simulink model "ZT_VehCtrl_18B"  (R2018b)
settings: Solver=FixedStepAuto  StartTime=0.0  StopTime=inf  FixedStep=0.005  RelTol=1e-3
InitFcn:
  | mbd_mpc_consistency_checks(bdroot(gcs));
undefined symbols (not defined in the file or in its folder): ANG_DEAD, BMS_NormalPwr, BrkPrsByBrkPct_TB_X, BrkPrsByBrkPct_TB_Y, DELAY_DISCHARGE, DELAY_RCUOFF, DRV_BACKWARD, DRV_BRAKE, DRV_FORWARD, DRV_NEUTRAL, DRV_PARK, DRV_UNPARK, DRV_ZEROTURN, EPB_LOCK, EPB_UNLOCK, ExtraLoadPwr, FanOff, fifo_0_vect, fifo_1_vect, HiFanReq, HV_finished, HV_No_Active, HV_POWER_OFF, HV_POWER_ON, HVDown, HVON, KaTLS_v_DrgUp_X_VehSpd, KeFTM_s_Way1OffDlyTime, KeFTM_TK_Way1CoolLv2OffBatTemp, KeFTM_TK_Way1CoolLv2OffMtrTemp, KeFTM_TK_Way1CoolLv2OnBatTemp, KeFTM_TK_Way1CoolLv2OnMtrTemp, KeFTM_TK_Way1CoolLv3OffBatTemp, KeFTM_TK_Way1CoolLv3OffMtrTemp, KeFTM_TK_Way1CoolLv3OnBatTemp, KeFTM_TK_Way1CoolLv3OnMtrTemp, KeFTM_TK_Way1CoolLv4OffBatTemp, KeFTM_TK_Way1CoolLv4OffMtrTemp, KeFTM_TK_Way1CoolLv4OnBatTemp, KeFTM_TK_Way1CoolLv4OnMtrTemp, Kp1, Kp2, LowFanReq, LQFP, MtrPwrFactor_RCU, MtrPwrHighToMidThd, MtrPwrLowToMidThd, MtrPwrMidToHighThd, MtrPwrMidToLowThd, MtrTrqMax, PCT_DEAD, Precharge, PTO_1000, PTO_540, pts1_fifo_0_vect, pts1_fifo_1_vect, pts2_fifo_0_vect, pts2_fifo_1_vect, pts3_fifo_0_vect, pts3_fifo_1_vect ... (+24)
libraries: mbd_mpc574x_ec_toolbox x173, canmsglib x72, simulink x57
(part 6 of 12)

== system ZT_VehCtrl_18B/SigOut/GPIO /HS ==
  note: 3A/5A
  note: 1A/3A
  note: 0.5A/1A
  Data Store Read : DataStoreRead  DataStoreName=HS001
  Data Store Read2 : DataStoreRead  DataStoreName=HS007
  Data Store Read4 : DataStoreRead  DataStoreName=HS002
  Data Store Read5 : DataStoreRead  DataStoreName=HS003
  Data Store Read6 : DataStoreRead  DataStoreName=HS004
  Data Store Read7 : DataStoreRead  DataStoreName=HS005
  Data Store Read9 : DataStoreRead  DataStoreName=HS010
  HS001 : mbd_mpc574x_ec_toolbox/GPIO Blocks/Digital_Output  Priority=1  gpio_pin=PTF5: [SIUL2_GPIO85 | General Purpose IO PF[5]]  gpio_drive_strength=Disabled
  "HS002 " : mbd_mpc574x_ec_toolbox/GPIO Blocks/Digital_Output  Priority=1  gpio_pin=PTF4: [SIUL2_GPIO84 | General Purpose IO PF[4]]  gpio_drive_strength=Disabled
  HS003 : mbd_mpc574x_ec_toolbox/GPIO Blocks/Digital_Output  Priority=1  gpio_pin=PTF3: [SIUL2_GPIO83 | General Purpose IO PF[3]]  gpio_drive_strength=Disabled
  HS004 : mbd_mpc574x_ec_toolbox/GPIO Blocks/Digital_Output  Priority=1  gpio_pin=PTB6: [SIUL2_GPIO22 | General Purpose IO PB[6]]  gpio_drive_strength=Disabled
  HS005 : mbd_mpc574x_ec_toolbox/GPIO Blocks/Digital_Output  Priority=1  gpio_pin=PTA12: [SIUL2_GPIO12 | General Purpose IO PA[12]]  gpio_drive_strength=Disabled
  HS007 : mbd_mpc574x_ec_toolbox/GPIO Blocks/Digital_Output  Priority=1  gpio_pin=PTF7: [SIUL2_GPIO87 | General Purpose IO PF[7]]  gpio_drive_strength=Disabled
  HS010 : mbd_mpc574x_ec_toolbox/GPIO Blocks/Digital_Output  Priority=1  gpio_pin=PTF9: [SIUL2_GPIO89 | General Purpose IO PF[9]]  gpio_drive_strength=Disabled
  wires:
  Data Store Read/1 -> HS001/1
  Data Store Read5/1 -> HS003/1
  Data Store Read4/1 -> "HS002 "/1
  Data Store Read6/1 -> HS004/1
  Data Store Read7/1 -> HS005/1
  Data Store Read2/1 -> HS007/1
  Data Store Read9/1 -> HS010/1

== system ZT_VehCtrl_18B/SigOut/GPIO /PWM_OUT ==
  note: LS PWM
  note: HS PWM
  note: Example
  Data Store Read10 : DataStoreRead  DataStoreName=HSO14_PWM_DC
  Data Store Read11 : DataStoreRead  DataStoreName=HSO14_PWM_FRQ
  Data Store Read14 : DataStoreRead  DataStoreName=LSO19_PWM_DC
  Data Store Read15 : DataStoreRead  DataStoreName=LSO19_PWM_FRQ
  Data Store Read2 : DataStoreRead  DataStoreName=HSO08_PWM_DC
  Data Store Read9 : DataStoreRead  DataStoreName=HSO08_PWM_FRQ
  FreqCMD : Stateflow chart  Priority=0  Commented=on  TreatAsAtomicUnit=on
  PWM Configuration and Frequency Update : Subsystem  Commented=on
  PWM Configuration and Frequency Update1 : Subsystem
  PWM Configuration and Frequency Update4 : Subsystem
  wires:
  FreqCMD/1(freq) -> PWM Configuration and Frequency Update/1(In1)
  FreqCMD/2(dc) -> PWM Configuration and Frequency Update/2(In2)
  Data Store Read9/1 -> PWM Configuration and Frequency Update1/2(Fre A)
  Data Store Read2/1 -> PWM Configuration and Frequency Update1/1(PWM A)
  Data Store Read14/1 -> PWM Configuration and Frequency Update4/1(PWM A)
  Data Store Read10/1 -> PWM Configuration and Frequency Update1/3(PWM B)
  Data Store Read11/1 -> PWM Configuration and Frequency Update1/4(Fre B)
  Data Store Read15/1 -> PWM Configuration and Frequency Update4/2(Fre)

== system ZT_VehCtrl_18B/SigOut/GPIO /SPI0: LS09_14_15_16_1_2_11_4 ==
  note: 不要开，会重置SPI的初始化设置
  Compare To Constant : simulink/Logic and Bit Operations/Compare To Constant  relop===  const=2  OutDataTypeStr=boolean
  Constant : Constant  OutDataTypeStr=boolean
  Constant1 : Constant  OutDataTypeStr=boolean
  Constant2 : Constant  OutDataTypeStr=boolean
  Data Store Read : DataStoreRead  DataStoreName=VCU_Mode
  Data Store Read1 : DataStoreRead  DataStoreName=SPI0_CS
  LS_CTRL : Subsystem
  LS_CTRL1 : Subsystem
  LS_EN : mbd_mpc574x_ec_toolbox/GPIO Blocks/Digital_Output  Priority=1  gpio_pin=PTA2: [SIUL2_GPIO2 | General Purpose IO PA[2]]  gpio_drive_strength=Disabled
  LS_rst1 : mbd_mpc574x_ec_toolbox/GPIO Blocks/Digital_Output  Priority=1  gpio_pin=PTC10: [SIUL2_GPIO42 | General Purpose IO PC[10]]  gpio_drive_strength=Disabled
  LS_rst2 : mbd_mpc574x_ec_toolbox/GPIO Blocks/Digital_Output  Priority=1  gpio_pin=PTA1: [SIUL2_GPIO1 | General Purpose IO PA[1]]  gpio_drive_strength=Disabled
  Logical Operator : Logic  AllPortsSameDT=off  OutDataTypeStr=boolean
  Logical Operator1 : Logic  Operator=NOT  AllPortsSameDT=off  OutDataTypeStr=boolean
  wires:
  Constant1/1 -> LS_rst2/1
  Constant/1 -> LS_EN/1
  Constant2/1 -> LS_rst1/1
  Data Store Read/1 -> Compare To Constant/1
  Compare To Constant/1 -> Logical Operator/1
  Data Store Read1/1 -> Logical Operator/2
  Logical Operator/1 -> LS_CTRL1/Enable, Logical Operator1/1
  Logical Operator1/1 -> LS_CTRL/Enable

== system ZT_VehCtrl_18B/SigOut/GPIO /SPI3: LS03_06_07_08_10_12_13_17_18_19 ==
  Compare To Constant : simulink/Logic and Bit Operations/Compare To Constant  relop===  const=2  OutDataTypeStr=boolean
  Constant1 : Constant  OutDataTypeStr=boolean
  Constant3 : Constant  OutDataTypeStr=boolean
  Data Store Read : DataStoreRead  DataStoreName=VCU_Mode
  Data Store Read3 : DataStoreRead  DataStoreName=SPI3_CS
  LS_EN1 : mbd_mpc574x_ec_toolbox/GPIO Blocks/Digital_Output  Priority=1  gpio_pin=PTF10: [SIUL2_GPIO90 | General Purpose IO PF[10]]  gpio_drive_strength=Disabled
  LS_rst : mbd_mpc574x_ec_toolbox/GPIO Blocks/Digital_Output  Priority=1  gpio_pin=PTC14: [SIUL2_GPIO46 | General Purpose IO PC[14]]  gpio_drive_strength=Disabled
  Logical Operator : Logic  AllPortsSameDT=off  OutDataTypeStr=boolean
  Subsystem : Subsystem
  wires:
  Constant1/1 -> LS_EN1/1
  Constant3/1 -> LS_rst/1
  Data Store Read/1 -> Compare To Constant/1
  Data Store Read3/1 -> Logical Operator/2
  Compare To Constant/1 -> Logical Operator/1
  Logical Operator/1 -> Subsystem/Enable

== system ZT_VehCtrl_18B/VehCtrl/EnergyManage1/Subsystem ==
  VehTrqTgt : Inport
  VehSpd : Inport  Port=2
  MCU_PTO : Inport  Port=3
  Add : Sum
  Bus Selector3 : BusSelector  OutputSignals=MCU2VCU_1.MCU_TrqEst,MCU2VCU_1.MCU_SpdEst
  Constant2 : Constant  Value=WhlRadius
  Constant3 : Constant  Value=9.55  OutDataTypeStr=single
  Divide : Product  Inputs=*/
  Divide1 : Product  Inputs=*/
  Product : Product
  Product1 : Product
  PwrCmd : Outport
  wires:
  Constant3/1 -> Divide1/2
  Divide/1 -> Product/2
  Product/1 -> Add/1
  Constant2/1 -> Divide/2
  Bus Selector3/2 -> Divide1/1  "<MCU_SpdEst>"
  Divide1/1 -> Product1/2
  Product1/1 -> Add/2
  Bus Selector3/1 -> Product1/1  "<MCU_TrqEst>"
  VehTrqTgt/1 -> Product/1
  VehSpd/1 -> Divide/1
  Add/1 -> PwrCmd/1
  MCU_PTO/1 -> Bus Selector3/1

== system ZT_VehCtrl_18B/VehCtrl/FaultProc/Subsystem5 ==
  note: 1-正常
      | 0-超时
  note: 1-丢包
      | 0-正常
  AutoDrive : Inport
  Bus Selector7 : BusSelector  OutputSignals=signal1.AUTO_LiveCnt1,signal1.AUTO_CheckSum1,signal1.PacketLossFlg,signal2.AUTO_LiveCnt2,signal2.AUTO_CheckSum2,signal2.PacketLossFlg,signal3.AUTO_LiveCnt1,signal3.AUTO_CheckSum1,signal3.PacketLossFlg
  Logical Operator : Logic  Operator=NOT  AllPortsSameDT=off  OutDataTypeStr=boolean
  Logical Operator1 : Logic  Operator=OR  Inputs=3  AllPortsSameDT=off  OutDataTypeStr=boolean
  Logical Operator2 : Logic  Inputs=3  AllPortsSameDT=off  OutDataTypeStr=boolean
  PacketLoss_RMT : Stateflow chart  TreatAsAtomicUnit=on
  PacketLoss_RMT1 : Stateflow chart  TreatAsAtomicUnit=on
  PacketLoss_RMT2 : Stateflow chart  TreatAsAtomicUnit=on
  TimeOutLevel_RMT : Stateflow chart  TreatAsAtomicUnit=on
  TimeOutLevel_RMT1 : Stateflow chart  TreatAsAtomicUnit=on
  TimeOutLevel_RMT2 : Stateflow chart  TreatAsAtomicUnit=on
  TimeOut : Outport
  PacketLoss : Outport  Port=2
  wires:
  TimeOutLevel_RMT/1(TimeOutLevel) -> Logical Operator2/1  "TimeOutLevel1"
  Logical Operator2/1 -> Logical Operator/1
  [Auto_LiveCounter] -> TimeOutLevel_RMT/1(LiveCounter)
  Logical Operator1/1 -> PacketLoss/1
  [Auto_PacketLossFlg] -> PacketLoss_RMT/2(PacketLoss)
  [Auto_CheckSumFlg] -> PacketLoss_RMT/1(CheckSum)
  PacketLoss_RMT/1(PacketLossFlg) -> Logical Operator1/1
  AutoDrive/1 -> Bus Selector7/1
  Logical Operator/1 -> TimeOut/1
  [Auto_LiveCounter2] -> TimeOutLevel_RMT1/1(LiveCounter)
  TimeOutLevel_RMT1/1(TimeOutLevel) -> Logical Operator2/2  "TimeOutLevel1"
  [Auto_CheckSumFlg2] -> PacketLoss_RMT1/1(CheckSum)
  [Auto_PacketLossFlg2] -> PacketLoss_RMT1/2(PacketLoss)
  PacketLoss_RMT1/1(PacketLossFlg) -> Logical Operator1/2
  Bus Selector7/6 -> [Auto_PacketLossFlg2]  "<PacketLossFlg>"
  Bus Selector7/5 -> [Auto_CheckSumFlg2]  "<AUTO_CheckSum2>"
  Bus Selector7/4 -> [Auto_LiveCounter2]  "<AUTO_LiveCnt2>"
  Bus Selector7/3 -> [Auto_PacketLossFlg]  "<PacketLossFlg>"
  Bus Selector7/2 -> [Auto_CheckSumFlg]  "<AUTO_CheckSum1>"
  Bus Selector7/1 -> [Auto_LiveCounter]  "<AUTO_LiveCnt1>"
  Bus Selector7/7 -> [Auto_LiveCounter3]  "<AUTO_LiveCnt1>"
  Bus Selector7/8 -> [Auto_CheckSumFlg3]  "<AUTO_CheckSum1>"
  Bus Selector7/9 -> [Auto_PacketLossFlg3]  "<PacketLossFlg>"
  [Auto_LiveCounter3] -> TimeOutLevel_RMT2/1(LiveCounter)
  TimeOutLevel_RMT2/1(TimeOutLevel) -> Logical Operator2/3  "TimeOutLevel1"
  [Auto_PacketLossFlg3] -> PacketLoss_RMT2/2(PacketLoss)
  [Auto_CheckSumFlg3] -> PacketLoss_RMT2/1(CheckSum)
  PacketLoss_RMT2/1(PacketLossFlg) -> Logical Operator1/3

== system ZT_VehCtrl_18B/VehCtrl/MontionControl/DriveControl ==
  EN_COM : Inport
  Ready : Inport  Port=2
  Fault : Inport  Port=3
  CMD : Inport  Port=4
  BMS : Inport  Port=5
  VehSpd : Inport  Port=6
  StrReady : Inport  Port=7
  AUTO : Inport  Port=8
  AUTOMode : Inport  Port=9
  RMT : Inport  Port=10
  DCDC : Inport  Port=11
  Brake : Subsystem
  Bus Creator{1..4} (4 alike) : BusCreator  Inputs=4
  Bus Selector : BusSelector  OutputSignals=RMT.RMT1.RMT_CmdAccPct,BrkPct,ModeDir,ModeStr,StrAng,RMT.RMT4.ModeSafety
  Constant : Constant  Value=0  OutDataTypeStr=uint8
  Constant1 : Constant
  Constant2 : Constant  Value=0  OutDataTypeStr=uint8
  Constant3 : Constant  OutDataTypeStr=boolean
  DriveModeTrans : Stateflow chart  TreatAsAtomicUnit=on
  Equal : RelationalOperator  Operator===  OutDataTypeStr=boolean  RndMeth=Simplest
  Logical Operator : Logic  AllPortsSameDT=off  OutDataTypeStr=boolean
  Motor : Subsystem
  MCUFL_OUT : Outport
  MCUFR_OUT : Outport  Port=2
  MCURL_OUT : Outport  Port=3
  MCURR_OUT : Outport  Port=4
  BrkPrsTgt : Outport  Port=5
  EpbSt : Outport  Port=6
  VehTrqTgt : Outport  Port=7
  wires:
  CMD/1 -> Bus Selector/1
  Bus Selector/3 -> DriveModeTrans/5(ModeDirection)  "<ModeDir>"
  Bus Selector/2 -> DriveModeTrans/2(CmdBrk)  "<BrkPct>"
  Brake/1(BrkPrsTgt) -> BrkPrsTgt/1
  DriveModeTrans/1(VehBrk) -> Brake/1(VehBrkTgt)
  DriveModeTrans/2(EpbSt) -> EpbSt/1
  VehSpd/1 -> DriveModeTrans/9(VehSpd), Motor/5(VehSpd)
  DriveModeTrans/3(VehDrv) -> Motor/1(VehDrvPct)
  Bus Selector/1 -> DriveModeTrans/1(CmdDrv)  "<RMT_CmdAccPct>"
  Bus Selector/4 -> Logical Operator/1  "<ModeStr>"
  StrReady/1 -> DriveModeTrans/8(StrReady)
  DriveModeTrans/4(SpdTgt) -> Motor/2(CmdSpd)
  DriveModeTrans/5(ModeSpd) -> Motor/3(ModeSpeed)
  DriveModeTrans/6(DrvPhase) -> Motor/4(DrvPhase)
  Bus Selector/5 -> Motor/6(CmdStrAng)  "<StrAng>"
  Motor/2(MtrDirCmdFL) -> Bus Creator1/2  "DirCmd"
  Motor/1(Enable) -> Bus Creator1/1, Bus Creator2/1, Bus Creator4/1, Bus Creator3/1  "Enable"
  Bus Creator4/1 -> MCURR_OUT/1
  Bus Creator2/1 -> MCUFR_OUT/1
  Motor/13(MtrSpdCmdRR) -> Bus Creator4/4  "SpdCmd"
  Motor/12(MtrTrqCmdRR) -> Bus Creator4/3  "TrqCmd"
  Motor/11(MtrDirCmdRR) -> Bus Creator4/2  "DirCmd"
  Bus Creator1/1 -> MCUFL_OUT/1
  Motor/7(MtrSpdCmdFR) -> Bus Creator2/4  "SpdCmd"
  Motor/6(MtrTrqCmdFR) -> Bus Creator2/3  "TrqCmd"
  Bus Creator3/1 -> MCURL_OUT/1
  Motor/10(MtrSpdCmdRL) -> Bus Creator3/4  "SpdCmd"
  Motor/4(MtrSpdCmdFL) -> Bus Creator1/4  "SpdCmd"
  Motor/9(MtrTrqCmdRL) -> Bus Creator3/3  "TrqCmd"
  Motor/3(MtrTrqCmdFL) -> Bus Creator1/3  "TrqCmd"
  Motor/8(MtrDirCmdRL) -> Bus Creator3/2  "DirCmd"
  Motor/5(MtrDirCmdFR) -> Bus Creator2/2  "DirCmd"
  Ready/1 -> Motor/9(Ready)
  Motor/14(VehTrqTgt) -> VehTrqTgt/1
  Constant/1 -> DriveModeTrans/3(ModeDrive)
  Constant1/1 -> DriveModeTrans/4(CmdPark)
  Constant2/1 -> DriveModeTrans/7(CmdSpd)
  Bus Selector/6 -> Equal/1, Motor/7(ModeSafety)  "<ModeSafety>"
  AUTO/1 -> Motor/10(AUTO)
  AUTOMode/1 -> Motor/11(AUTOMode)
  BMS/1 -> Motor/12(BMS)
  RMT/1 -> Motor/13(RMT)
  DCDC/1 -> Motor/14(DCDC)
  Fault/1 -> Brake/2(In2), Motor/8(Fault)
  Logical Operator/1 -> DriveModeTrans/6(ModeSteer)
  Equal/1 -> Logical Operator/2
  Constant3/1 -> Equal/2
  EN_COM/1 -> Motor/15(EN_COM)

== system ZT_VehCtrl_18B/VehCtrl/MontionControl/PtoControl ==
  CMD : Inport
  Fault : Inport  Port=2
  Ready : Inport  Port=3
  AUTOMode : Inport  Port=4
  AUTO : Inport  Port=5
  Bus Creator : BusCreator  Inputs=4
  Bus Selector : BusSelector  OutputSignals=ShutDown,NonDrive,NonPto
  Bus Selector1 : BusSelector  OutputSignals=RMT.RMT4.RMT_PtoMode
  Bus Selector2 : BusSelector  OutputSignals=signal2.AUTO_PtoSpd
  Constant5 : Constant  Value=0  OutDataTypeStr=single
  Constant6 : Constant  OutDataTypeStr=uint8
  Constant7 : Constant  Value=0  OutDataTypeStr=uint8
  Logical Operator : Logic  Operator=OR  Inputs=3  AllPortsSameDT=off  OutDataTypeStr=boolean
  Logical Operator1 : Logic  AllPortsSameDT=off  OutDataTypeStr=boolean
  NOT : Logic  Operator=NOT  IconShape=distinctive  AllPortsSameDT=off  OutDataTypeStr=boolean
  Subsystem : Subsystem
  Subsystem1 : Subsystem
  Switch2 : Switch  Criteria=u2 > Threshold
  MCU_PTO_OUT : Outport
  wires:
  CMD/1 -> Bus Selector1/1
  Constant5/1 -> Bus Creator/3  "MtrTrqCmd"
  Subsystem/1(ModeReq) -> Bus Creator/1  "ModeReq"
  Constant6/1 -> Subsystem/1(ModeSpeed)
  Constant7/1 -> Subsystem/2(DirCmd)
  Fault/1 -> Bus Selector/1
  Bus Selector/1 -> Logical Operator/1  "<ShutDown>"
  Bus Selector/2 -> Logical Operator/2  "<NonDrive>"
  Bus Selector/3 -> Logical Operator/3  "<NonPto>"
  Logical Operator/1 -> NOT/1
  Ready/1 -> Logical Operator1/2
  NOT/1 -> Logical Operator1/1
  Logical Operator1/1 -> Bus Creator/4  "Enable"
  Bus Creator/1 -> MCU_PTO_OUT/1
  AUTOMode/1 -> Switch2/2
  Bus Selector1/1 -> Subsystem1/1(<RMT_PtoMode>)  "<RMT_PtoMode>"
  AUTO/1 -> Bus Selector2/1
  Bus Selector2/1 -> Switch2/1  "<AUTO_PtoSpd>"
  Switch2/1 -> Bus Creator/2  "MtrSpdCmd"
  Subsystem1/1(MtrSpdCmd) -> Switch2/3

== system ZT_VehCtrl_18B/VehCtrl/MontionControl/SteerControl ==
  note: 这个是模式，不是方向
  VehSpd : Inport
  CMD : Inport  Port=2
  BDX : Inport  Port=3
  Bus Selector : BusSelector  OutputSignals=ModeStr,StrAng
  Bus Selector1 : BusSelector  OutputSignals=AVCU.BDX_SteeringAngle
  Chart : Stateflow chart  TreatAsAtomicUnit=on
  Constant2 : Constant  Value=10  OutDataTypeStr=uint8
  GreaterThan : RelationalOperator  Operator=<  OutDataTypeStr=boolean  RndMeth=Simplest
  StrReady : Outport
  AngCmd : Outport  Port=2
  wires:
  CMD/1 -> Bus Selector/1
  Bus Selector/1 -> Chart/2(Mode)  "<ModeStr>"
  Bus Selector/2 -> Chart/3(AngCmd)  "<StrAng>"
  BDX/1 -> Bus Selector1/1
  Bus Selector1/1 -> Chart/4(Ang)  "<BDX_SteeringAngle>"
  Chart/2(StrPhase) -> GreaterThan/1
  GreaterThan/1 -> StrReady/1
  Constant2/1 -> GreaterThan/2
  VehSpd/1 -> Chart/1(VehSpd)
  Chart/1(AngCmdOut) -> AngCmd/1

== system ZT_VehCtrl_18B/VehCtrl/MontionControl/ValveControl ==
  note: 仅在安全模式下才能控制
  BrkPrsTgt : Inport
  EpbSt : Inport  Port=2
  BDX : Inport  Port=3
  CMD : Inport  Port=4
  Ready : Inport  Port=5
  "AngCmd " : Inport  Port=6
  fault : Inport  Port=7
  VehSpd : Inport  Port=8
  BrakeSys : Subsystem
  Bus Creator : BusCreator  Inputs=9
  Bus Selector : BusSelector  OutputSignals=ModeSusp,RMT.RMT4.ModeSafety,RMT.RMT2.RMT_ModeWidth
  Bus Selector1 : BusSelector  OutputSignals=AVCU.BDX_BrakePressure
  Bus Selector2 : BusSelector  OutputSignals=NonDrive
  EpbSys : Subsystem
  PumpSys : Subsystem
  SteerSys : Subsystem
  SuspesionSys : Subsystem
  WidthSys : Subsystem
  BDX_OUT : Outport
  wires:
  CMD/1 -> Bus Selector/1
  BDX/1 -> Bus Selector1/1
  BrkPrsTgt/1 -> BrakeSys/1(BrkPrsTgt)
  Bus Selector1/1 -> BrakeSys/2(BrkPrs)  "<BDX_BrakePressure>"
  Bus Selector/1 -> SuspesionSys/1(SuspSt)  "<ModeSusp>"
  Bus Selector/3 -> WidthSys/2(<RMT_ModeWidth>)  "<RMT_ModeWidth>"
  BrakeSys/1(BrkValve) -> Bus Creator/2  "BrkValve"
  SuspesionSys/1(SuspUpValve) -> Bus Creator/6  "SuspUpValve"
  PumpSys/1(Pump) -> Bus Creator/1  "Pump"
  EpbSys/1(EpbValve) -> Bus Creator/5  "EpbValve"
  SteerSys/1(SteerValveL) -> Bus Creator/3  "SteerValveL"
  WidthSys/1(WidthLengthenValve) -> Bus Creator/8  "WidthLengthenValve"
  WidthSys/2(WidthShortenValve) -> Bus Creator/9  "WidthShortenValve"
  Bus Creator/1 -> BDX_OUT/1
  SteerSys/2(SteerValveR) -> Bus Creator/4  "SteerValveR"
  EpbSt/1 -> EpbSys/1(EpbSt)
  SuspesionSys/2(SuspDownValve) -> Bus Creator/7  "SuspDownValve"
  Ready/1 -> PumpSys/1(Ready)
  Bus Selector/2 -> WidthSys/1(ModeSafety), SuspesionSys/2(ModeSafety)  "<ModeSafety>"
  fault/1 -> Bus Selector2/1
  Bus Selector2/1 -> SteerSys/2(In2)  "<NonDrive>"
  VehSpd/1 -> SteerSys/3(VehSpd)
  "AngCmd "/1 -> SteerSys/1(AngCmd)

== system ZT_VehCtrl_18B/VehCtrl/TempertureControl/Lv_to_Dut1 ==
  note: 就是整型，不要替换为single
  MCUReqMtrPumpLv : Inport
  2-D Lookup Table1 : Lookup_n-D  NumberOfTableDimensions=1  BreakpointsForDimension1=uint8([ 0 1 2 3 4 ])  BreakpointsForDimension2=KaTLS_v_DrgUp_X_VehSpd  Table=uint16([ 5 30 40 55 70])  TableDataTypeStr=uint16  ExtrapMethod=Clip  UseLastTableValue=on  OutDataTypeStr=Inherit: Inherit from 'Table data'  RndMeth=Simplest
  Gain : Gain  Gain=1/100  OutDataTypeStr=single
  MCUReqMtrPumpDut : Outport
  wires:
  MCUReqMtrPumpLv/1 -> 2-D Lookup Table1/1
  2-D Lookup Table1/1 -> Gain/1
  Gain/1 -> MCUReqMtrPumpDut/1

== system ZT_VehCtrl_18B/VehCtrl/TempertureControl/Lv_to_Dut2 ==
  note: 就是整型，不要替换为single
  MCUReqMtrPumpLv : Inport
  2-D Lookup Table1 : Lookup_n-D  NumberOfTableDimensions=1  BreakpointsForDimension1=uint8([ 0 1 2 3 4 ])  BreakpointsForDimension2=KaTLS_v_DrgUp_X_VehSpd  Table=uint16([ 5 30 40 55 70])  TableDataTypeStr=uint16  ExtrapMethod=Clip  UseLastTableValue=on  OutDataTypeStr=Inherit: Inherit from 'Table data'  RndMeth=Simplest
  Gain : Gain  Gain=1/100  OutDataTypeStr=single
  MCUReqMtrPumpDut : Outport
  wires:
  MCUReqMtrPumpLv/1 -> 2-D Lookup Table1/1
  2-D Lookup Table1/1 -> Gain/1
  Gain/1 -> MCUReqMtrPumpDut/1

== system ZT_VehCtrl_18B/VehCtrl/TempertureControl/Lv_to_Dut3 ==
  note: 就是整型，不要替换为single
  MCUReqBatPumpLv : Inport
  2-D Lookup Table1 : Lookup_n-D  NumberOfTableDimensions=1  BreakpointsForDimension1=uint8([ 0 1 2 3 4 ])  BreakpointsForDimension2=KaTLS_v_DrgUp_X_VehSpd  Table=uint16([ 5 30 40 55 70])  TableDataTypeStr=uint16  ExtrapMethod=Clip  UseLastTableValue=on  OutDataTypeStr=Inherit: Inherit from 'Table data'  RndMeth=Simplest
  Gain : Gain  Gain=1/100  OutDataTypeStr=single
  MCUReqBatPumpDut : Outport
  wires:
  MCUReqBatPumpLv/1 -> 2-D Lookup Table1/1
  2-D Lookup Table1/1 -> Gain/1
  Gain/1 -> MCUReqBatPumpDut/1

== system ZT_VehCtrl_18B/VehCtrl/TempertureControl/ThermFR_RRvRead1 ==
  RdySt : Inport
  MtrTemp : Inport  Port=2
  Cnt_To_s : Subsystem
  Constant10 : Constant  Value=KeFTM_TK_Way1CoolLv3OnMtrTemp
  Constant11 : Constant  Value=KeFTM_TK_Way1CoolLv2OffMtrTemp
  Constant12 : Constant  Value=KeFTM_TK_Way1CoolLv2OnMtrTemp
  Constant13 : Constant  Value=KeFTM_TK_Way1CoolLv4OnMtrTemp
  Constant7 : Constant  Value=KeFTM_s_Way1OffDlyTime
  Constant8 : Constant  Value=KeFTM_TK_Way1CoolLv4OffMtrTemp
  Constant9 : Constant  Value=KeFTM_TK_Way1CoolLv3OffMtrTemp
  Way1_Cool_Level : Stateflow chart  TreatAsAtomicUnit=on
  MtrPumpLvReq : Outport
  Fan_Low : Outport  Port=2
  wires:
  Way1_Cool_Level/2(MtrPumpLv) -> MtrPumpLvReq/1  "MtrPumpLvReq2"
  Way1_Cool_Level/1(Fan_Low) -> Fan_Low/1  "FanLvReq2"
  RdySt/1 -> Way1_Cool_Level/1(RdySt)
  Constant13/1 -> Way1_Cool_Level/8(Ke_Lv4OnTemp)
  Constant12/1 -> Way1_Cool_Level/4(Ke_Lv2OnTemp)
  Constant10/1 -> Way1_Cool_Level/6(Ke_Lv3OnTemp)
  Constant9/1 -> Way1_Cool_Level/5(Ke_Lv3OffTemp)
  Constant11/1 -> Way1_Cool_Level/3(Ke_Lv2OffTemp)
  Constant7/1 -> Cnt_To_s/1(In1)
  Constant8/1 -> Way1_Cool_Level/7(Ke_Lv4OffTemp)
  Cnt_To_s/1(Out1) -> Way1_Cool_Level/9(Ke_OffDlyCnt)
  MtrTemp/1 -> Way1_Cool_Level/2(Temp)

== system ZT_VehCtrl_18B/VehCtrl/TempertureControl/ThermFR_RRvRead2 ==
  RdySt : Inport
  MtrTemp : Inport  Port=2
  Cnt_To_s : Subsystem
  Constant10 : Constant  Value=KeFTM_TK_Way1CoolLv3OnMtrTemp
  Constant11 : Constant  Value=KeFTM_TK_Way1CoolLv2OffMtrTemp
  Constant12 : Constant  Value=KeFTM_TK_Way1CoolLv2OnMtrTemp
  Constant13 : Constant  Value=KeFTM_TK_Way1CoolLv4OnMtrTemp
  Constant7 : Constant  Value=KeFTM_s_Way1OffDlyTime
  Constant8 : Constant  Value=KeFTM_TK_Way1CoolLv4OffMtrTemp
  Constant9 : Constant  Value=KeFTM_TK_Way1CoolLv3OffMtrTemp
  Way1_Cool_Level : Stateflow chart  TreatAsAtomicUnit=on
  MtrPumpLvReq : Outport
  Fan_Low : Outport  Port=2
  wires:
  MtrTemp/1 -> Way1_Cool_Level/2(Temp)
  Cnt_To_s/1(Out1) -> Way1_Cool_Level/9(Ke_OffDlyCnt)
  Constant8/1 -> Way1_Cool_Level/7(Ke_Lv4OffTemp)
  Constant7/1 -> Cnt_To_s/1(In1)
  Constant11/1 -> Way1_Cool_Level/3(Ke_Lv2OffTemp)
  Constant9/1 -> Way1_Cool_Level/5(Ke_Lv3OffTemp)
  Constant10/1 -> Way1_Cool_Level/6(Ke_Lv3OnTemp)
  Constant12/1 -> Way1_Cool_Level/4(Ke_Lv2OnTemp)
  Constant13/1 -> Way1_Cool_Level/8(Ke_Lv4OnTemp)
  RdySt/1 -> Way1_Cool_Level/1(RdySt)
  Way1_Cool_Level/1(Fan_Low) -> Fan_Low/1  "FanLvReq2"
  Way1_Cool_Level/2(MtrPumpLv) -> MtrPumpLvReq/1  "MtrPumpLvReq2"

== system ZT_VehCtrl_18B/VehCtrl/TempertureControl/ThermLvRead3 ==
  RdySt : Inport
  Temp : Inport  Port=2
  Cnt_To_s : Subsystem
  Constant10 : Constant  Value=KeFTM_TK_Way1CoolLv3OnBatTemp
  Constant11 : Constant  Value=KeFTM_TK_Way1CoolLv2OffBatTemp
  Constant12 : Constant  Value=KeFTM_TK_Way1CoolLv2OnBatTemp
  Constant13 : Constant  Value=KeFTM_TK_Way1CoolLv4OnBatTemp
  Constant7 : Constant  Value=KeFTM_s_Way1OffDlyTime
  Constant8 : Constant  Value=KeFTM_TK_Way1CoolLv4OffBatTemp
  Constant9 : Constant  Value=KeFTM_TK_Way1CoolLv3OffBatTemp
  Way1_Cool_Level : Stateflow chart  TreatAsAtomicUnit=on
  Fan_Low : Outport
  Fan_High : Outport  Port=2
  v1 : Outport  Port=3
  v2 : Outport  Port=4
  v3 : Outport  Port=5
  v4 : Outport  Port=6
  PumpLvReq : Outport  Port=7
  wires:
  Way1_Cool_Level/2(Fan_High) -> Fan_High/1
  Temp/1 -> Way1_Cool_Level/2(Temp)
  RdySt/1 -> Way1_Cool_Level/1(RdySt)
  Constant13/1 -> Way1_Cool_Level/8(Ke_Lv4OnTemp)
  Constant9/1 -> Way1_Cool_Level/5(Ke_Lv3OffTemp)
  Constant12/1 -> Way1_Cool_Level/4(Ke_Lv2OnTemp)
  Constant10/1 -> Way1_Cool_Level/6(Ke_Lv3OnTemp)
  Constant7/1 -> Cnt_To_s/1(In1)
  Constant8/1 -> Way1_Cool_Level/7(Ke_Lv4OffTemp)
  Cnt_To_s/1(Out1) -> Way1_Cool_Level/9(Ke_OffDlyCnt)
  Constant11/1 -> Way1_Cool_Level/3(Ke_Lv2OffTemp)
  Way1_Cool_Level/7(MtrPumpLv) -> PumpLvReq/1  "MtrPumpLvReq2"
  Way1_Cool_Level/1(Fan_Low) -> Fan_Low/1  "FanLvReq2"
  Way1_Cool_Level/3(V1) -> v1/1
  Way1_Cool_Level/4(V2) -> v2/1
  Way1_Cool_Level/5(V3) -> v3/1
  Way1_Cool_Level/6(V4) -> v4/1

== system ZT_VehCtrl_18B/Initialization & SPI timer1/CS1 LS/Subsystem/SPI_en ==
  Action Port : ActionPort
  Add : Sum
  Add1 : Sum  Inputs=+++
  Constant1 : Constant  Value=0
  Constant11 : Constant  OutDataTypeStr=uint8
  Constant2 : Constant  OutDataTypeStr=uint8
  Constant3 : Constant  Value=0
  Constant9 : Constant  Value=128  OutDataTypeStr=uint8
  Data Type Conversion : DataTypeConversion
  Data Type Conversion1 : DataTypeConversion
  Gain : Gain  Gain=64
  Out1 : Outport
  Out2 : Outport  Port=2
  wires:
  Constant1/1 -> Add/1
  Constant9/1 -> Add1/1
  Add1/1 -> Data Type Conversion/1
  Constant11/1 -> Add1/2
  Constant2/1 -> Gain/1
  Gain/1 -> Add1/3
  Add/1 -> Data Type Conversion1/1
  Constant3/1 -> Add/2
  Data Type Conversion/1 -> Out1/1
  Data Type Conversion1/1 -> Out2/1

== system ZT_VehCtrl_18B/Initialization & SPI timer1/CS1 LS/Subsystem/clear  ==
  Action Port : ActionPort
  Add : Sum
  Add1 : Sum  Inputs=+++
  Constant1 : Constant
  Constant11 : Constant  Value=7  OutDataTypeStr=uint8
  Constant2 : Constant  Value=0  OutDataTypeStr=uint8
  Constant3 : Constant  Value=0
  Constant9 : Constant  Value=128  OutDataTypeStr=uint8
  Data Type Conversion : DataTypeConversion
  Data Type Conversion1 : DataTypeConversion
  Gain : Gain  Gain=64
  Out1 : Outport
  Out2 : Outport  Port=2
  wires:
  Constant3/1 -> Add/2
  Add/1 -> Data Type Conversion1/1
  Gain/1 -> Add1/3
  Constant2/1 -> Gain/1
  Constant11/1 -> Add1/2
  Add1/1 -> Data Type Conversion/1
  Data Type Conversion1/1 -> Out2/1
  Data Type Conversion/1 -> Out1/1
  Constant9/1 -> Add1/1
  Constant1/1 -> Add/1

== system ZT_VehCtrl_18B/Initialization & SPI timer1/CS1 LS/Subsystem/confi_enbit ==
  Action Port : ActionPort
  Add : Sum
  Add1 : Sum  Inputs=+++
  Constant1 : Constant
  Constant11 : Constant  Value=7  OutDataTypeStr=uint8
  Constant2 : Constant  OutDataTypeStr=uint8
  Constant3 : Constant  Value=128
  Constant9 : Constant  Value=128  OutDataTypeStr=uint8
  Data Type Conversion : DataTypeConversion
  Data Type Conversion1 : DataTypeConversion
  Gain : Gain  Gain=64
  Out1 : Outport
  Out2 : Outport  Port=2
  wires:
  Constant1/1 -> Add/1
  Constant9/1 -> Add1/1
  Add1/1 -> Data Type Conversion/1
  Constant11/1 -> Add1/2
  Constant2/1 -> Gain/1
  Gain/1 -> Add1/3
  Add/1 -> Data Type Conversion1/1
  Constant3/1 -> Add/2
  Data Type Conversion/1 -> Out1/1
  Data Type Conversion1/1 -> Out2/1

== system ZT_VehCtrl_18B/Initialization & SPI timer1/CS3 LS/Subsystem/A组配置 ==
  Action Port : ActionPort
  Add : Sum  Inputs=+++
  Add1 : Sum  Inputs=+++
  Bias : Bias  Bias=1
  Constant : Constant
  Constant10 : Constant  Value=2
  Constant9 : Constant  Value=80  OutDataTypeStr=uint8
  Data Store Read1 : DataStoreRead  DataStoreName=cnt2
  Data Store Write : DataStoreWrite  DataStoreName=SPI3_CTRL1
  Data Store Write1 : DataStoreWrite  DataStoreName=cnt2
  Data Type Conversion : DataTypeConversion  OutDataTypeStr=uint8
  Data Type Conversion1 : DataTypeConversion  OutDataTypeStr=uint8
  Data Type Conversion2 : DataTypeConversion
  Gain : Gain  Gain=4
  Gain1 : Gain
  Gain2 : Gain  Gain=4
  Gain3 : Gain
  Manual Switch : ManualSwitch  CurrentSetting=0
  PIN : Constant  Value=2
  SPI : Constant  Value=0
  Switch4 : Switch  Criteria=u2 > Threshold  Threshold=2
  default SPI : Constant  Value=0
  Out1 : Outport  VectorParamsAs1DForOutWhenUnconnected=on
  Out2 : Outport  Port=2  VectorParamsAs1DForOutWhenUnconnected=on
  wires:
  Switch4/1 -> Data Type Conversion2/1
  Constant/1 -> Switch4/3
  Constant10/1 -> Switch4/1
  Data Store Read1/1 -> Bias/1
  Bias/1 -> Data Store Write1/1, Switch4/2
  Data Type Conversion2/1 -> Data Store Write/1
  Data Type Conversion/1 -> Out1/1
  Data Type Conversion1/1 -> Out2/1
  Constant9/1 -> Add1/1
  Add/1 -> Data Type Conversion1/1
  [Mode] -> Gain3/1, Gain2/1, Gain1/1, Gain/1
  Gain2/1 -> Add/1
  Gain3/1 -> Add/2
  default SPI/1 -> Add/3
  Add1/1 -> Data Type Conversion/1
  Gain/1 -> Add1/2
  Gain1/1 -> Add1/3
  SPI/1 -> Manual Switch/1
  Manual Switch/1 -> [Mode]
  PIN/1 -> Manual Switch/2

== system ZT_VehCtrl_18B/Initialization & SPI timer1/CS3 LS/Subsystem/B组配置 ==
  Action Port : ActionPort
  Bias : Bias  Bias=1
  Constant : Constant  Value=2
  Constant1 : Constant  Value=0  OutDataTypeStr=uint8
  Constant10 : Constant  Value=3
  Constant9 : Constant  Value=96  OutDataTypeStr=uint8
  Data Store Read1 : DataStoreRead  DataStoreName=cnt2
  Data Store Write : DataStoreWrite  DataStoreName=SPI3_CTRL1
  Data Store Write1 : DataStoreWrite  DataStoreName=cnt2
  Data Type Conversion : DataTypeConversion  OutDataTypeStr=uint8
  Data Type Conversion1 : DataTypeConversion  OutDataTypeStr=uint8
  Data Type Conversion2 : DataTypeConversion
  Switch4 : Switch  Criteria=u2 > Threshold  Threshold=4
  Out1 : Outport  VectorParamsAs1DForOutWhenUnconnected=on
  Out2 : Outport  Port=2  VectorParamsAs1DForOutWhenUnconnected=on
  wires:
  Data Type Conversion2/1 -> Data Store Write/1
  Bias/1 -> Switch4/2, Data Store Write1/1
  Data Store Read1/1 -> Bias/1
  Constant10/1 -> Switch4/1
  Constant/1 -> Switch4/3
  Switch4/1 -> Data Type Conversion2/1
  Constant1/1 -> Data Type Conversion1/1
  Data Type Conversion/1 -> Out1/1
  Constant9/1 -> Data Type Conversion/1
  Data Type Conversion1/1 -> Out2/1

== system ZT_VehCtrl_18B/Initialization & SPI timer1/CS5 LS/Subsystem/SPI_en ==
  Action Port : ActionPort
  Add : Sum
  Add1 : Sum  Inputs=+++
  Constant1 : Constant  Value=0
  Constant11 : Constant  OutDataTypeStr=uint8
  Constant2 : Constant  OutDataTypeStr=uint8
  Constant3 : Constant  Value=0
  Constant9 : Constant  Value=128  OutDataTypeStr=uint8
  Data Type Conversion : DataTypeConversion
  Data Type Conversion1 : DataTypeConversion
  Gain : Gain  Gain=64
  Out1 : Outport
  Out2 : Outport  Port=2
  wires:
  Constant1/1 -> Add/1
  Constant9/1 -> Add1/1
  Add1/1 -> Data Type Conversion/1
  Constant11/1 -> Add1/2
  Constant2/1 -> Gain/1
  Gain/1 -> Add1/3
  Add/1 -> Data Type Conversion1/1
  Constant3/1 -> Add/2
  Data Type Conversion/1 -> Out1/1
  Data Type Conversion1/1 -> Out2/1

== system ZT_VehCtrl_18B/Initialization & SPI timer1/CS5 LS/Subsystem/clear  ==
  Action Port : ActionPort
  Add : Sum
  Add1 : Sum  Inputs=+++
  Constant1 : Constant
  Constant11 : Constant  Value=7  OutDataTypeStr=uint8
  Constant2 : Constant  Value=0  OutDataTypeStr=uint8
  Constant3 : Constant  Value=0
  Constant9 : Constant  Value=128  OutDataTypeStr=uint8
  Data Type Conversion : DataTypeConversion
  Data Type Conversion1 : DataTypeConversion
  Gain : Gain  Gain=64
  Out1 : Outport
  Out2 : Outport  Port=2
  wires:
  Constant3/1 -> Add/2
  Add/1 -> Data Type Conversion1/1
  Gain/1 -> Add1/3
  Constant2/1 -> Gain/1
  Constant11/1 -> Add1/2
  Add1/1 -> Data Type Conversion/1
  Data Type Conversion1/1 -> Out2/1
  Data Type Conversion/1 -> Out1/1
  Constant9/1 -> Add1/1
  Constant1/1 -> Add/1

== system ZT_VehCtrl_18B/Initialization & SPI timer1/CS5 LS/Subsystem/confi_enbit ==
  Action Port : ActionPort
  Add : Sum
  Add1 : Sum  Inputs=+++
  Constant1 : Constant
  Constant11 : Constant  Value=7  OutDataTypeStr=uint8
  Constant2 : Constant  OutDataTypeStr=uint8
  Constant3 : Constant  Value=128
  Constant9 : Constant  Value=128  OutDataTypeStr=uint8
  Data Type Conversion : DataTypeConversion
  Data Type Conversion1 : DataTypeConversion
  Gain : Gain  Gain=64
  Out1 : Outport
  Out2 : Outport  Port=2
  wires:
  Constant1/1 -> Add/1
  Constant9/1 -> Add1/1
  Add1/1 -> Data Type Conversion/1
  Constant11/1 -> Add1/2
  Constant2/1 -> Gain/1
  Gain/1 -> Add1/3
  Add/1 -> Data Type Conversion1/1
  Constant3/1 -> Add/2
  Data Type Conversion/1 -> Out1/1
  Data Type Conversion1/1 -> Out2/1

== system ZT_VehCtrl_18B/SigIn/CAN0 /BMS Cell Battery Temperature/UNPACK ==
  ID : Inport
  data : Inport  Port=2
  length : Inport  Port=3
  timestamp : Inport  Port=4
  Action Port : ActionPort  ActionType=case
  Bus Creator : BusCreator  Inputs=7  OutDataTypeStr=Bus: CAN_MESSAGE_BUS  NonVirtualBus=on
  Bus Creator1 : BusCreator  Inputs=2
  CAN Unpack6 : canmsglib/CAN Unpack  CANdbFile=D:\VCU\VCU_SL_ZhengZhou\ZT2\模型与接口\CAN_DBC\整车CANA_GBK.dbc  MsgList=BMS_Cell_Battery_Temperature  MsgName=BMS_Cell_Battery_Temperature  MsgIDType=Standard (11-bit identifier)  MsgIdentifier=855  MsgLength=8  SignalInfo=CellTempearture_T1$16$8$2$2$1$0$1$-50$-50$125$#CellTempearture_T2$24$8$2$2$1$0$1$-50$-50$125$#CellTempearture_T3$32$8$2$2$1$0$1$-50$-50$125$#CellTempearture_T4$40$8$2$2$1$0$1$-50$-50$125$#CellTempearture_T5$48$8$2$2$1$0$1$-50$-50$125$#CellTempearture_T6$56$8$2$2$1$0$1$-50$-50$125$#CellTemperature_StartNum$8$16$2$2$1$0$1$0$0$1000$#  NSignals=7  IDPort=off  TimestampPort=off  ErrorPort=off  RemotePort=off  LengthPort=off  StatusPort=off  StartBits=str2num('[int32(16);int32(24);int32(32);int32(40);int32(48);int32(56);int32(8)]')  SignalSizes=str2num('[int32(8);int32(8);int32(8);int32(8);int32(8);int32(8);int32(16)]')  ByteOrders=str2num('[int32(2);int32(2);int32(2);int32(2);int32(2);int32(2);int32(2)]')  DataTypes=str2num('[int32(2);int32(2);int32(2);int32(2);int32(2);int32(2);int32(2)]')  MultiplexTypes=str2num('[int32(1);int32(1);int32(1);int32(1);int32(1);int32(1);int32(1)]')  MultiplexValues=str2num('[double(0);double(0);double(0);double(0);double(0);double(0);double(0)]')  Factors=str2num('[double(1);double(1);double(1);double(1);double(1);double(1);double(1)]')  Offsets=str2num('[double(-50);double(-50);double(-50);double(-50);double(-50);double(-50);double(0)]')  Minimums=str2num('[double(-50);double(-50);double(-50);double(-50);double(-50);double(-50);double(0)]')  Maximums=str2num('[double(125);double(125);double(125);double(125);double(125);double(125);double(1000)]')  ApplyMinMax=off
      settings: SourceProductName=Simulink Real-Time  SourceProductBaseCode=XP  DataFormat=CANdb specified signals
  Constant1 : Constant  Value=0  OutDataTypeStr=uint8
  Constant4 : Constant  Value=0  OutDataTypeStr=uint8
  Constant5 : Constant  Value=0  OutDataTypeStr=uint8
  Data Type Conversion{,14..15,17} (4 alike) : DataTypeConversion  OutDataTypeStr=uint8
  Data Type Conversion18 : DataTypeConversion  OutDataTypeStr=uint32
  Data Type Conversion19 : DataTypeConversion  OutDataTypeStr=double
  Message : Outport
  wires:
  Bus Creator1/1 -> Message/1
  Data Type Conversion15/1 -> Bus Creator/3  "Remote"
  Data Type Conversion14/1 -> Bus Creator/2  "Length"
  Data Type Conversion/1 -> Bus Creator/1  "Extended"
  Bus Creator/1 -> CAN Unpack6/1  "CAN_Msg_In"
  Data Type Conversion17/1 -> Bus Creator/4  "Error"
  timestamp/1 -> Data Type Conversion19/1
  Data Type Conversion19/1 -> Bus Creator/6  "Timestamp"
  ID/1 -> Data Type Conversion18/1
  Constant5/1 -> Data Type Conversion17/1
  Constant1/1 -> Data Type Conversion/1
  Data Type Conversion18/1 -> Bus Creator/5  "ID"
  data/1 -> Bus Creator/7  "Data"
  length/1 -> Data Type Conversion14/1
  Constant4/1 -> Data Type Conversion15/1

== system ZT_VehCtrl_18B/SigIn/CAN0 /BMS Cell HeatingTemperature/UNPACK ==
  ID : Inport
  data : Inport  Port=2
  length : Inport  Port=3
  timestamp : Inport  Port=4
  Action Port : ActionPort
  Bus Creator : BusCreator  Inputs=7  OutDataTypeStr=Bus: CAN_MESSAGE_BUS  NonVirtualBus=on
  Bus Creator1 : BusCreator  Inputs=2
  CAN Unpack6 : canmsglib/CAN Unpack  CANdbFile=D:\VCU\VCU_SL_ZhengZhou\ZT2\模型与接口\CAN_DBC\整车CANA_GBK.dbc  MsgList=BMS_Cell_HeatingTemperature  MsgName=BMS_Cell_HeatingTemperature  MsgIDType=Standard (11-bit identifier)  MsgIdentifier=1011  MsgLength=8  SignalInfo=CellHeatingTempearture_T1$16$8$2$2$1$0$1$-50$-50$125$#CellHeatingTempearture_T2$24$8$2$2$1$0$1$-50$-50$125$#CellHeatingTempearture_T3$32$8$2$2$1$0$1$-50$-50$125$#CellHeatingTempearture_T4$40$8$2$2$1$0$1$-50$-50$125$#CellHeatingTempearture_T5$48$8$2$2$1$0$1$-50$-50$125$#CellHeatingTempearture_T6$56$8$2$2$1$0$1$-50$-50$125$#CellHeatingTemperature_StartNum$8$16$2$2$1$0$1$0$0$1000$#  NSignals=7  IDPort=off  TimestampPort=off  ErrorPort=off  RemotePort=off  LengthPort=off  StatusPort=off  StartBits=str2num('[int32(16);int32(24);int32(32);int32(40);int32(48);int32(56);int32(8)]')  SignalSizes=str2num('[int32(8);int32(8);int32(8);int32(8);int32(8);int32(8);int32(16)]')  ByteOrders=str2num('[int32(2);int32(2);int32(2);int32(2);int32(2);int32(2);int32(2)]')  DataTypes=str2num('[int32(2);int32(2);int32(2);int32(2);int32(2);int32(2);int32(2)]')  MultiplexTypes=str2num('[int32(1);int32(1);int32(1);int32(1);int32(1);int32(1);int32(1)]')  MultiplexValues=str2num('[double(0);double(0);double(0);double(0);double(0);double(0);double(0)]')  Factors=str2num('[double(1);double(1);double(1);double(1);double(1);double(1);double(1)]')  Offsets=str2num('[double(-50);double(-50);double(-50);double(-50);double(-50);double(-50);double(0)]')  Minimums=str2num('[double(-50);double(-50);double(-50);double(-50);double(-50);double(-50);double(0)]')  Maximums=str2num('[double(125);double(125);double(125);double(125);double(125);double(125);double(1000)]')  ApplyMinMax=off
      settings: SourceProductName=Simulink Real-Time  SourceProductBaseCode=XP  DataFormat=CANdb specified signals
  Constant1 : Constant  Value=0  OutDataTypeStr=uint8
  Constant4 : Constant  Value=0  OutDataTypeStr=uint8
  Constant5 : Constant  Value=0  OutDataTypeStr=uint8
  Data Type Conversion{,14..15,17} (4 alike) : DataTypeConversion  OutDataTypeStr=uint8
  Data Type Conversion18 : DataTypeConversion  OutDataTypeStr=uint32
  Data Type Conversion19 : DataTypeConversion  OutDataTypeStr=double
  Message : Outport
  wires:
  Constant4/1 -> Data Type Conversion15/1
  length/1 -> Data Type Conversion14/1
  data/1 -> Bus Creator/7  "Data"
  Data Type Conversion18/1 -> Bus Creator/5  "ID"
  Constant1/1 -> Data Type Conversion/1
  Constant5/1 -> Data Type Conversion17/1
  ID/1 -> Data Type Conversion18/1
  Data Type Conversion19/1 -> Bus Creator/6  "Timestamp"
  timestamp/1 -> Data Type Conversion19/1
  Data Type Conversion17/1 -> Bus Creator/4  "Error"
  Bus Creator/1 -> CAN Unpack6/1  "CAN_Msg_In"
  Data Type Conversion/1 -> Bus Creator/1  "Extended"
  Data Type Conversion14/1 -> Bus Creator/2  "Length"
  Data Type Conversion15/1 -> Bus Creator/3  "Remote"
  Bus Creator1/1 -> Message/1

== system ZT_VehCtrl_18B/SigIn/CAN0 /BMS Cell Pole Temperature/UNPACK ==
  ID : Inport
  data : Inport  Port=2
  length : Inport  Port=3
  timestamp : Inport  Port=4
  Action Port : ActionPort
  Bus Creator : BusCreator  Inputs=7  OutDataTypeStr=Bus: CAN_MESSAGE_BUS  NonVirtualBus=on
  Bus Creator1 : BusCreator  Inputs=2
  CAN Unpack6 : canmsglib/CAN Unpack  CANdbFile=D:\VCU\VCU_SL_ZhengZhou\ZT2\模型与接口\CAN_DBC\整车CANA_GBK.dbc  MsgList=BMS_Cell_Pole_Temperature  MsgName=BMS_Cell_Pole_Temperature  MsgIDType=Standard (11-bit identifier)  MsgIdentifier=1012  MsgLength=8  SignalInfo=CellPoleTempearture_T1$16$8$2$2$1$0$1$-50$-50$125$#CellPoleTempearture_T2$24$8$2$2$1$0$1$-50$-50$125$#CellPoleTempearture_T3$32$8$2$2$1$0$1$-50$-50$125$#CellPoleTempearture_T4$40$8$2$2$1$0$1$-50$-50$125$#CellPoleTempearture_T5$48$8$2$2$1$0$1$-50$-50$125$#CellPoleTempearture_T6$56$8$2$2$1$0$1$-50$-50$125$#CellPoleTemperature_StartNum$8$16$2$2$1$0$1$0$0$1000$#  NSignals=7  IDPort=off  TimestampPort=off  ErrorPort=off  RemotePort=off  LengthPort=off  StatusPort=off  StartBits=str2num('[int32(16);int32(24);int32(32);int32(40);int32(48);int32(56);int32(8)]')  SignalSizes=str2num('[int32(8);int32(8);int32(8);int32(8);int32(8);int32(8);int32(16)]')  ByteOrders=str2num('[int32(2);int32(2);int32(2);int32(2);int32(2);int32(2);int32(2)]')  DataTypes=str2num('[int32(2);int32(2);int32(2);int32(2);int32(2);int32(2);int32(2)]')  MultiplexTypes=str2num('[int32(1);int32(1);int32(1);int32(1);int32(1);int32(1);int32(1)]')  MultiplexValues=str2num('[double(0);double(0);double(0);double(0);double(0);double(0);double(0)]')  Factors=str2num('[double(1);double(1);double(1);double(1);double(1);double(1);double(1)]')  Offsets=str2num('[double(-50);double(-50);double(-50);double(-50);double(-50);double(-50);double(0)]')  Minimums=str2num('[double(-50);double(-50);double(-50);double(-50);double(-50);double(-50);double(0)]')  Maximums=str2num('[double(125);double(125);double(125);double(125);double(125);double(125);double(1000)]')  ApplyMinMax=off
      settings: SourceProductName=Simulink Real-Time  SourceProductBaseCode=XP  DataFormat=CANdb specified signals
  Constant1 : Constant  Value=0  OutDataTypeStr=uint8
  Constant4 : Constant  Value=0  OutDataTypeStr=uint8
  Constant5 : Constant  Value=0  OutDataTypeStr=uint8
  Data Type Conversion{,14..15,17} (4 alike) : DataTypeConversion  OutDataTypeStr=uint8
  Data Type Conversion18 : DataTypeConversion  OutDataTypeStr=uint32
  Data Type Conversion19 : DataTypeConversion  OutDataTypeStr=double
  Message : Outport
  wires:
  Bus Creator1/1 -> Message/1
  Data Type Conversion15/1 -> Bus Creator/3  "Remote"
  Data Type Conversion14/1 -> Bus Creator/2  "Length"
  Data Type Conversion/1 -> Bus Creator/1  "Extended"
  Bus Creator/1 -> CAN Unpack6/1  "CAN_Msg_In"
  Data Type Conversion17/1 -> Bus Creator/4  "Error"
  timestamp/1 -> Data Type Conversion19/1
  Data Type Conversion19/1 -> Bus Creator/6  "Timestamp"
  ID/1 -> Data Type Conversion18/1
  Constant5/1 -> Data Type Conversion17/1
  Constant1/1 -> Data Type Conversion/1
  Data Type Conversion18/1 -> Bus Creator/5  "ID"
  data/1 -> Bus Creator/7  "Data"
  length/1 -> Data Type Conversion14/1
  Constant4/1 -> Data Type Conversion15/1

== system ZT_VehCtrl_18B/SigIn/CAN0 /BMS Cell Voltage Infor/UNPACK ==
  ID : Inport
  data : Inport  Port=2
  length : Inport  Port=3
  timestamp : Inport  Port=4
  Action Port : ActionPort  ActionType=case
  Bus Creator : BusCreator  Inputs=7  OutDataTypeStr=Bus: CAN_MESSAGE_BUS  NonVirtualBus=on
  Bus Creator1 : BusCreator  Inputs=4
  CAN Unpack6 : canmsglib/CAN Unpack  CANdbFile=D:\VCU\VCU_SL_ZhengZhou\ZT2\模型与接口\CAN_DBC\整车CANA_GBK.dbc  MsgList=BMS_Cell_Voltage_Infor  MsgName=BMS_Cell_Voltage_Infor  MsgIDType=Standard (11-bit identifier)  MsgIdentifier=854  MsgLength=8  SignalInfo=CellVoltage_StartNum$8$16$2$2$1$0$1$0$0$1000$#CellVoltage_V1$24$16$2$2$1$0$1.000000e-03$0$0$10$#CellVoltage_V2$40$16$2$2$1$0$1.000000e-03$0$0$10$#CellVoltage_V3$56$16$2$2$1$0$1.000000e-03$0$0$10$#  NSignals=4  IDPort=off  TimestampPort=off  ErrorPort=off  RemotePort=off  LengthPort=off  StatusPort=off  StartBits=str2num('[int32(8);int32(24);int32(40);int32(56)]')  SignalSizes=str2num('[int32(16);int32(16);int32(16);int32(16)]')  ByteOrders=str2num('[int32(2);int32(2);int32(2);int32(2)]')  DataTypes=str2num('[int32(2);int32(2);int32(2);int32(2)]')  MultiplexTypes=str2num('[int32(1);int32(1);int32(1);int32(1)]')  MultiplexValues=str2num('[double(0);double(0);double(0);double(0)]')  Factors=str2num('[double(1);double(1.000000e-03);double(1.000000e-03);double(1.000000e-03)]')  Offsets=str2num('[double(0);double(0);double(0);double(0)]')  Minimums=str2num('[double(0);double(0);double(0);double(0)]')  Maximums=str2num('[double(1000);double(10);double(10);double(10)]')  ApplyMinMax=off
      settings: SourceProductName=Simulink Real-Time  SourceProductBaseCode=XP  DataFormat=CANdb specified signals
  Constant1 : Constant  Value=0  OutDataTypeStr=uint8
  Constant4 : Constant  Value=0  OutDataTypeStr=uint8
  Constant5 : Constant  Value=0  OutDataTypeStr=uint8
  Data Type Conversion{,14..15,17} (4 alike) : DataTypeConversion  OutDataTypeStr=uint8
  Data Type Conversion18 : DataTypeConversion  OutDataTypeStr=uint32
  Data Type Conversion19 : DataTypeConversion  OutDataTypeStr=double
  Message : Outport
  wires:
  Bus Creator1/1 -> Message/1
  Data Type Conversion15/1 -> Bus Creator/3  "Remote"
  Data Type Conversion14/1 -> Bus Creator/2  "Length"
  Data Type Conversion/1 -> Bus Creator/1  "Extended"
  Bus Creator/1 -> CAN Unpack6/1  "CAN_Msg_In"
  Data Type Conversion17/1 -> Bus Creator/4  "Error"
  timestamp/1 -> Data Type Conversion19/1
  Data Type Conversion19/1 -> Bus Creator/6  "Timestamp"
  ID/1 -> Data Type Conversion18/1
  Constant5/1 -> Data Type Conversion17/1
  Constant1/1 -> Data Type Conversion/1
  Data Type Conversion18/1 -> Bus Creator/5  "ID"
  data/1 -> Bus Creator/7  "Data"
  length/1 -> Data Type Conversion14/1
  Constant4/1 -> Data Type Conversion15/1

== system ZT_VehCtrl_18B/SigIn/CAN0 /BMS CumuCap Infor/UNPACK ==
  ID : Inport
  data : Inport  Port=2
  length : Inport  Port=3
  timestamp : Inport  Port=4
  Action Port : ActionPort
  Bus Creator : BusCreator  Inputs=7  OutDataTypeStr=Bus: CAN_MESSAGE_BUS  NonVirtualBus=on
  Bus Creator1 : BusCreator  Inputs=2
  CAN Unpack6 : canmsglib/CAN Unpack  CANdbFile=D:\VCU\VCU_SL_ZhengZhou\ZT2\模型与接口\CAN_DBC\整车CANA_GBK.dbc  MsgList=BMS_CumuCap_Infor  MsgName=BMS_CumuCap_Infor  MsgIDType=Standard (11-bit identifier)  MsgIdentifier=1013  MsgLength=8  SignalInfo=CumuCap_Charge$56$32$2$2$1$0$1$0$0$4294967295$#CumuCap_Discharge$24$32$2$2$1$0$1$0$0$4294967295$#  NSignals=2  IDPort=off  TimestampPort=off  ErrorPort=off  RemotePort=off  LengthPort=off  StatusPort=off  StartBits=str2num('[int32(56);int32(24)]')  SignalSizes=str2num('[int32(32);int32(32)]')  ByteOrders=str2num('[int32(2);int32(2)]')  DataTypes=str2num('[int32(2);int32(2)]')  MultiplexTypes=str2num('[int32(1);int32(1)]')  MultiplexValues=str2num('[double(0);double(0)]')  Factors=str2num('[double(1);double(1)]')  Offsets=str2num('[double(0);double(0)]')  Minimums=str2num('[double(0);double(0)]')  Maximums=str2num('[double(4294967295);double(4294967295)]')  ApplyMinMax=off
      settings: SourceProductName=Simulink Real-Time  SourceProductBaseCode=XP  DataFormat=CANdb specified signals
  Constant1 : Constant  Value=0  OutDataTypeStr=uint8
  Constant4 : Constant  Value=0  OutDataTypeStr=uint8
  Constant5 : Constant  Value=0  OutDataTypeStr=uint8
  Data Type Conversion{,14..15,17} (4 alike) : DataTypeConversion  OutDataTypeStr=uint8
  Data Type Conversion18 : DataTypeConversion  OutDataTypeStr=uint32
  Data Type Conversion19 : DataTypeConversion  OutDataTypeStr=double
  Message : Outport
  wires:
  Constant4/1 -> Data Type Conversion15/1
  length/1 -> Data Type Conversion14/1
  data/1 -> Bus Creator/7  "Data"
  Data Type Conversion18/1 -> Bus Creator/5  "ID"
  Constant1/1 -> Data Type Conversion/1
  Constant5/1 -> Data Type Conversion17/1
  ID/1 -> Data Type Conversion18/1
  Data Type Conversion19/1 -> Bus Creator/6  "Timestamp"
  timestamp/1 -> Data Type Conversion19/1
  Data Type Conversion17/1 -> Bus Creator/4  "Error"
  Bus Creator/1 -> CAN Unpack6/1  "CAN_Msg_In"
  Data Type Conversion/1 -> Bus Creator/1  "Extended"
  Data Type Conversion14/1 -> Bus Creator/2  "Length"
  Data Type Conversion15/1 -> Bus Creator/3  "Remote"
  Bus Creator1/1 -> Message/1

== system ZT_VehCtrl_18B/SigIn/CAN0 /BMS CumuTimeInfor1/UNPACK ==
  ID : Inport
  data : Inport  Port=2
  length : Inport  Port=3
  timestamp : Inport  Port=4
  Action Port : ActionPort
  Bus Creator : BusCreator  Inputs=7  OutDataTypeStr=Bus: CAN_MESSAGE_BUS  NonVirtualBus=on
  Bus Creator1 : BusCreator  Inputs=2
  CAN Unpack6 : canmsglib/CAN Unpack  CANdbFile=D:\VCU\VCU_SL_ZhengZhou\ZT2\模型与接口\CAN_DBC\整车CANA_GBK.dbc  MsgList=BMS_CumuTimeInfor1  MsgName=BMS_CumuTimeInfor1  MsgIDType=Standard (11-bit identifier)  MsgIdentifier=515  MsgLength=8  SignalInfo=CumuTime_Charge$56$32$2$2$1$0$1.000000e-01$0$0$4294967295$#CumuTime_Discharge$24$32$2$2$1$0$1.000000e-01$0$0$4294967295$#  NSignals=2  IDPort=off  TimestampPort=off  ErrorPort=off  RemotePort=off  LengthPort=off  StatusPort=off  StartBits=str2num('[int32(56);int32(24)]')  SignalSizes=str2num('[int32(32);int32(32)]')  ByteOrders=str2num('[int32(2);int32(2)]')  DataTypes=str2num('[int32(2);int32(2)]')  MultiplexTypes=str2num('[int32(1);int32(1)]')  MultiplexValues=str2num('[double(0);double(0)]')  Factors=str2num('[double(1.000000e-01);double(1.000000e-01)]')  Offsets=str2num('[double(0);double(0)]')  Minimums=str2num('[double(0);double(0)]')  Maximums=str2num('[double(4294967295);double(4294967295)]')  ApplyMinMax=off
      settings: SourceProductName=Simulink Real-Time  SourceProductBaseCode=XP  DataFormat=CANdb specified signals
  Constant1 : Constant  Value=0  OutDataTypeStr=uint8
  Constant4 : Constant  Value=0  OutDataTypeStr=uint8
  Constant5 : Constant  Value=0  OutDataTypeStr=uint8
  Data Type Conversion{,14..15,17} (4 alike) : DataTypeConversion  OutDataTypeStr=uint8
  Data Type Conversion18 : DataTypeConversion  OutDataTypeStr=uint32
  Data Type Conversion19 : DataTypeConversion  OutDataTypeStr=double
  Message : Outport
  wires:
  Bus Creator1/1 -> Message/1
  Data Type Conversion15/1 -> Bus Creator/3  "Remote"
  Data Type Conversion14/1 -> Bus Creator/2  "Length"
  Data Type Conversion/1 -> Bus Creator/1  "Extended"
  Bus Creator/1 -> CAN Unpack6/1  "CAN_Msg_In"
  Data Type Conversion17/1 -> Bus Creator/4  "Error"
  timestamp/1 -> Data Type Conversion19/1
  Data Type Conversion19/1 -> Bus Creator/6  "Timestamp"
  ID/1 -> Data Type Conversion18/1
  Constant5/1 -> Data Type Conversion17/1
  Constant1/1 -> Data Type Conversion/1
  Data Type Conversion18/1 -> Bus Creator/5  "ID"
  data/1 -> Bus Creator/7  "Data"
  length/1 -> Data Type Conversion14/1
  Constant4/1 -> Data Type Conversion15/1
